simulink model "PX4_Run_Mode_R2016b"  (R2017b)
settings: Solver=FixedStepDiscrete  StartTime=0.0  StopTime=inf  FixedStep=Ts  RelTol=1e-3  EnableMultiTasking=on
InitFcn:
  | run('InitFcn_R2016b.m');
values from neighbouring files (symbols this model uses):
  A = Pixhawk_CSC.Parameter( {single([diag([1 1 1]) Ts*diag([1 1 1]); diag([0 0 0]) diag([1 1 1])]),'A'} )    [InitFcn.m]    (also in InitFcn_R2016b.m; InitFcn_R2017b_no_csc.m = single([diag([1 1 1]) Ts*diag([1 1 1]); diag([0 0 0]) diag([)
  app = Pixhawk_CSC.Parameter({single( [0.05; 0.05; 0.05]),'app'} )    [InitFcn.m]    (also in InitFcn_R2016b.m; InitFcn_R2017b_no_csc.m = single( [0.05; 0.05; 0.05]))
  B = Pixhawk_CSC.Parameter( {single([Ts^2/2*diag([1 1 1]); Ts*diag([1 1 1])]),'B'} )    [InitFcn.m]    (also in InitFcn_R2016b.m; InitFcn_R2017b_no_csc.m = single([Ts^2/2*diag([1 1 1]); Ts*diag([1 1 1])]))
  Beta = Pixhawk_CSC.Parameter({single( 0.02),'Beta'} )    [InitFcn.m]    (also in InitFcn_R2016b.m; InitFcn_R2017b_no_csc.m = single( 0.02))
  C = Pixhawk_CSC.Parameter( {single([diag([1 1 1]) 0*diag([1 1 1]); zeros(1,2) 1 zeros(1,3)]),'C'} )    [InitFcn.m]    (also in InitFcn_R2016b.m; InitFcn_R2017b_no_csc.m = single([diag([1 1 1]) 0*diag([1 1 1]); zeros(1,2) 1 zeros(1,)
  C1 = Pixhawk_CSC.Parameter({single( 1.08680),'C1'} )    [InitFcn.m]    (also in InitFcn_R2016b.m; InitFcn_R2017b_no_csc.m = single( 1.08680))
  C10 = Pixhawk_CSC.Parameter({single( 0.0000),'C10'} )    [InitFcn.m]    (also in InitFcn_R2016b.m; InitFcn_R2017b_no_csc.m = single( 0.0000))
  C11 = Pixhawk_CSC.Parameter({single(-0.2300),'C11'} )    [InitFcn.m]    (also in InitFcn_R2016b.m; InitFcn_R2017b_no_csc.m = single(-0.2300))
  C12 = Pixhawk_CSC.Parameter({single( 0.0000),'C12'} )    [InitFcn.m]    (also in InitFcn_R2016b.m; InitFcn_R2017b_no_csc.m = single( 0.0000))
  C13 = Pixhawk_CSC.Parameter({single( 0.8000),'C13'} )    [InitFcn.m]    (also in InitFcn_R2016b.m; InitFcn_R2017b_no_csc.m = single( 0.8000))
  C14 = Pixhawk_CSC.Parameter({single( 0.8000),'C14'} )    [InitFcn.m]    (also in InitFcn_R2016b.m; InitFcn_R2017b_no_csc.m = single( 0.8000))
  C15 = Pixhawk_CSC.Parameter({single( 1.73200),'C15'} )    [InitFcn.m]    (also in InitFcn_R2016b.m; InitFcn_R2017b_no_csc.m = single( 1.73200))
  C16 = Pixhawk_CSC.Parameter({single( 0.1000),'C16'} )    [InitFcn.m]    (also in InitFcn_R2016b.m; InitFcn_R2017b_no_csc.m = single( 0.1000))
  C17 = Pixhawk_CSC.Parameter({single( 0.1000),'C17'} )    [InitFcn.m]    (also in InitFcn_R2016b.m; InitFcn_R2017b_no_csc.m = single( 0.1000))
  C18 = Pixhawk_CSC.Parameter({single( 0.0500),'C18'} )    [InitFcn.m]    (also in InitFcn_R2016b.m; InitFcn_R2017b_no_csc.m = single( 0.0500))
  C19 = Pixhawk_CSC.Parameter({single( 0.6000),'C19'} )    [InitFcn.m]    (also in InitFcn_R2016b.m; InitFcn_R2017b_no_csc.m = single( 0.6000))
  C2 = Pixhawk_CSC.Parameter({single( 1.10468),'C2'} )    [InitFcn.m]    (also in InitFcn_R2016b.m; InitFcn_R2017b_no_csc.m = single( 1.10468))
  C20 = Pixhawk_CSC.Parameter({single( 0.6000),'C20'} )    [InitFcn.m]    (also in InitFcn_R2016b.m; InitFcn_R2017b_no_csc.m = single( 0.6000))
  C21 = Pixhawk_CSC.Parameter({single( 1.04558),'C21'} )    [InitFcn.m]    (also in InitFcn_R2016b.m; InitFcn_R2017b_no_csc.m = single( 1.04558))
  C22 = Pixhawk_CSC.Parameter({single( 0.0000),'C22'} )    [InitFcn.m]    (also in InitFcn_R2016b.m; InitFcn_R2017b_no_csc.m = single( 0.0000))
  C23 = Pixhawk_CSC.Parameter({single( 0.0000),'C23'} )    [InitFcn.m]    (also in InitFcn_R2016b.m; InitFcn_R2017b_no_csc.m = single( 0.0000))
  C24 = Pixhawk_CSC.Parameter({single(-11.0000),'C24'} )    [InitFcn.m]    (also in InitFcn_R2016b.m; InitFcn_R2017b_no_csc.m = single(-11.0000))
  C3 = Pixhawk_CSC.Parameter({single( 1.1980),'C3'} )    [InitFcn.m]    (also in InitFcn_R2016b.m; InitFcn_R2017b_no_csc.m = single( 1.1980))
  C4 = Pixhawk_CSC.Parameter({single( 0.0500),'C4'} )    [InitFcn.m]    (also in InitFcn_R2016b.m; InitFcn_R2017b_no_csc.m = single( 0.0500))
  C5 = Pixhawk_CSC.Parameter({single( 0.0500),'C5'} )    [InitFcn.m]    (also in InitFcn_R2016b.m; InitFcn_R2017b_no_csc.m = single( 0.0500))
  C6 = Pixhawk_CSC.Parameter({single( 0.0500),'C6'} )    [InitFcn.m]    (also in InitFcn_R2016b.m; InitFcn_R2017b_no_csc.m = single( 0.0500))
  C7 = Pixhawk_CSC.Parameter({single( 0.35937),'C7'} )    [InitFcn.m]    (also in InitFcn_R2016b.m; InitFcn_R2017b_no_csc.m = single( 0.35937))
  C8 = Pixhawk_CSC.Parameter({single( 0.36528),'C8'} )    [InitFcn.m]    (also in InitFcn_R2016b.m; InitFcn_R2017b_no_csc.m = single( 0.36528))
  C9 = Pixhawk_CSC.Parameter({single( 0.53311),'C9'} )    [InitFcn.m]    (also in InitFcn_R2016b.m; InitFcn_R2017b_no_csc.m = single( 0.53311))
  C_1 = Pixhawk_CSC.Parameter( {single([diag([1 1 1]) 0*diag([1 1 1])]),'C1'} )    [InitFcn.m]    (also in InitFcn_R2016b.m; InitFcn_R2017b_no_csc.m = single([diag([1 1 1]) 0*diag([1 1 1])]))
  CAL_ACC0_XOFFSET = Pixhawk_CSC.Parameter( {single( 0.122052  ),'CAL_ACC0_XOFFSET'} )    [InitFcn.m]    (also in InitFcn_R2016b.m; InitFcn_R2017b_no_csc.m = single( 0.122052  ))
  CAL_ACC0_XXSCALE = Pixhawk_CSC.Parameter( {single(  1.01218    ),'CAL_ACC0_XXSCALE'} )    [InitFcn.m]    (also in InitFcn_R2016b.m; InitFcn_R2017b_no_csc.m = single(  1.01218    ))
  CAL_ACC0_XYSCALE = Pixhawk_CSC.Parameter( {single( -0.00443301 ),'CAL_ACC0_XYSCALE'} )    [InitFcn.m]    (also in InitFcn_R2016b.m; InitFcn_R2017b_no_csc.m = single( -0.00443301 ))
  CAL_ACC0_XZSCALE = Pixhawk_CSC.Parameter( {single( -0.00505793 ),'CAL_ACC0_XZSCALE'} )    [InitFcn.m]    (also in InitFcn_R2016b.m; InitFcn_R2017b_no_csc.m = single( -0.00505793 ))
  CAL_ACC0_YOFFSET = Pixhawk_CSC.Parameter( {single( 0.00281205),'CAL_ACC0_YOFFSET'} )    [InitFcn.m]    (also in InitFcn_R2016b.m; InitFcn_R2017b_no_csc.m = single( 0.00281205))
  CAL_ACC0_YXSCALE = Pixhawk_CSC.Parameter( {single( -0.00443301 ),'CAL_ACC0_YXSCALE'} )    [InitFcn.m]    (also in InitFcn_R2016b.m; InitFcn_R2017b_no_csc.m = single( -0.00443301 ))
  CAL_ACC0_YYSCALE = Pixhawk_CSC.Parameter( {single(  1.00234    ),'CAL_ACC0_YYSCALE'} )    [InitFcn.m]    (also in InitFcn_R2016b.m; InitFcn_R2017b_no_csc.m = single(  1.00234    ))
  CAL_ACC0_YZSCALE = Pixhawk_CSC.Parameter( {single(  0.0160883  ),'CAL_ACC0_YZSCALE'} )    [InitFcn.m]    (also in InitFcn_R2016b.m; InitFcn_R2017b_no_csc.m = single(  0.0160883  ))
  CAL_ACC0_ZOFFSET = Pixhawk_CSC.Parameter( {single(-0.0298121 ),'CAL_ACC0_ZOFFSET'} )    [InitFcn.m]    (also in InitFcn_R2016b.m; InitFcn_R2017b_no_csc.m = single(-0.0298121 ))
  CAL_ACC0_ZXSCALE = Pixhawk_CSC.Parameter( {single( -0.00505793 ),'CAL_ACC0_ZXSCALE'} )    [InitFcn.m]    (also in InitFcn_R2016b.m; InitFcn_R2017b_no_csc.m = single( -0.00505793 ))
  CAL_ACC0_ZYSCALE = Pixhawk_CSC.Parameter( {single(  0.0160883  ),'CAL_ACC0_ZYSCALE'} )    [InitFcn.m]    (also in InitFcn_R2016b.m; InitFcn_R2017b_no_csc.m = single(  0.0160883  ))
  CAL_ACC0_ZZSCALE = Pixhawk_CSC.Parameter( {single(  0.983604   ),'CAL_ACC0_ZZSCALE'} )    [InitFcn.m]    (also in InitFcn_R2016b.m; InitFcn_R2017b_no_csc.m = single(  0.983604   ))
  CAL_BAR_OFFSET = Pixhawk_CSC.Parameter( {single( -20.8468),'CAL_BAR_OFFSET'} )    [InitFcn.m]    (also in InitFcn_R2016b.m; InitFcn_R2017b_no_csc.m = single( -20.8468))
  CAL_BAR_SCALE = Pixhawk_CSC.Parameter( {single(   1.0632),'CAL_BAR_SCALE'} )    [InitFcn.m]    (also in InitFcn_R2016b.m; InitFcn_R2017b_no_csc.m = single(   1.0632))
  CAL_BAT0_XOFFSET = Pixhawk_CSC.Parameter( {single( 0.0000),'CAL_BAT0_XOFFSET'} )    [InitFcn.m]    (also in InitFcn_R2016b.m; InitFcn_R2017b_no_csc.m = single( 0.0000))
  CAL_BAT0_XXSCALE = Pixhawk_CSC.Parameter( {single(  1.0000),'CAL_BAT0_XXSCALE'} )    [InitFcn.m]    (also in InitFcn_R2016b.m; InitFcn_R2017b_no_csc.m = single(  1.0000))
  CAL_BAT0_XYSCALE = Pixhawk_CSC.Parameter( {single(  0.0000),'CAL_BAT0_XYSCALE'} )    [InitFcn.m]    (also in InitFcn_R2016b.m; InitFcn_R2017b_no_csc.m = single(  0.0000))
  CAL_BAT0_XZSCALE = Pixhawk_CSC.Parameter( {single(  0.0000),'CAL_BAT0_XZSCALE'} )    [InitFcn.m]    (also in InitFcn_R2016b.m; InitFcn_R2017b_no_csc.m = single(  0.0000))
  CAL_BAT0_YOFFSET = Pixhawk_CSC.Parameter( {single( 0.0000),'CAL_BAT0_YOFFSET'} )    [InitFcn.m]    (also in InitFcn_R2016b.m; InitFcn_R2017b_no_csc.m = single( 0.0000))
  CAL_BAT0_YXSCALE = Pixhawk_CSC.Parameter( {single(  0.0000),'CAL_BAT0_YXSCALE'} )    [InitFcn.m]    (also in InitFcn_R2016b.m; InitFcn_R2017b_no_csc.m = single(  0.0000))
  CAL_BAT0_YYSCALE = Pixhawk_CSC.Parameter( {single(  1.0000),'CAL_BAT0_YYSCALE'} )    [InitFcn.m]    (also in InitFcn_R2016b.m; InitFcn_R2017b_no_csc.m = single(  1.0000))
  CAL_BAT0_YZSCALE = Pixhawk_CSC.Parameter( {single(  0.0000),'CAL_BAT0_YZSCALE'} )    [InitFcn.m]    (also in InitFcn_R2016b.m; InitFcn_R2017b_no_csc.m = single(  0.0000))
  CAL_BAT0_ZOFFSET = Pixhawk_CSC.Parameter( {single( 0.0000),'CAL_BAT0_ZOFFSET'} )    [InitFcn.m]    (also in InitFcn_R2016b.m; InitFcn_R2017b_no_csc.m = single( 0.0000))
  CAL_BAT0_ZXSCALE = Pixhawk_CSC.Parameter( {single(  0.0000),'CAL_BAT0_ZXSCALE'} )    [InitFcn.m]    (also in InitFcn_R2016b.m; InitFcn_R2017b_no_csc.m = single(  0.0000))
  CAL_BAT0_ZYSCALE = Pixhawk_CSC.Parameter( {single(  0.0000),'CAL_BAT0_ZYSCALE'} )    [InitFcn.m]    (also in InitFcn_R2016b.m; InitFcn_R2017b_no_csc.m = single(  0.0000))
  CAL_BAT0_ZZSCALE = Pixhawk_CSC.Parameter( {single(  1.0000),'CAL_BAT0_ZZSCALE'} )    [InitFcn.m]    (also in InitFcn_R2016b.m; InitFcn_R2017b_no_csc.m = single(  1.0000))
  CAL_GPS0_XOFFSET = Pixhawk_CSC.Parameter( {single( 0.0000),'CAL_GPS0_XOFFSET'} )    [InitFcn.m]    (also in InitFcn_R2016b.m; InitFcn_R2017b_no_csc.m = single( 0.0000))
  CAL_GPS0_XXSCALE = Pixhawk_CSC.Parameter( {single(  0.0100),'CAL_GPS0_XXSCALE'} )    [InitFcn.m]    (also in InitFcn_R2016b.m; InitFcn_R2017b_no_csc.m = single(  0.0100))
  CAL_GPS0_XYSCALE = Pixhawk_CSC.Parameter( {single(  0.0000),'CAL_GPS0_XYSCALE'} )    [InitFcn.m]    (also in InitFcn_R2016b.m; InitFcn_R2017b_no_csc.m = single(  0.0000))
  CAL_GPS0_XZSCALE = Pixhawk_CSC.Parameter( {single(  0.0000),'CAL_GPS0_XZSCALE'} )    [InitFcn.m]    (also in InitFcn_R2016b.m; InitFcn_R2017b_no_csc.m = single(  0.0000))
  CAL_GPS0_YOFFSET = Pixhawk_CSC.Parameter( {single( 0.0000),'CAL_GPS0_YOFFSET'} )    [InitFcn.m]    (also in InitFcn_R2016b.m; InitFcn_R2017b_no_csc.m = single( 0.0000))
  CAL_GPS0_YXSCALE = Pixhawk_CSC.Parameter( {single(  0.0000),'CAL_GPS0_YXSCALE'} )    [InitFcn.m]    (also in InitFcn_R2016b.m; InitFcn_R2017b_no_csc.m = single(  0.0000))
  CAL_GPS0_YYSCALE = Pixhawk_CSC.Parameter( {single(  0.0100),'CAL_GPS0_YYSCALE'} )    [InitFcn.m]    (also in InitFcn_R2016b.m; InitFcn_R2017b_no_csc.m = single(  0.0100))
  CAL_GPS0_YZSCALE = Pixhawk_CSC.Parameter( {single(  0.0000),'CAL_GPS0_YZSCALE'} )    [InitFcn.m]    (also in InitFcn_R2016b.m; InitFcn_R2017b_no_csc.m = single(  0.0000))
  CAL_GPS0_ZOFFSET = Pixhawk_CSC.Parameter( {single( 0.0000),'CAL_GPS0_ZOFFSET'} )    [InitFcn.m]    (also in InitFcn_R2016b.m; InitFcn_R2017b_no_csc.m = single( 0.0000))
  CAL_GPS0_ZXSCALE = Pixhawk_CSC.Parameter( {single(  0.0000),'CAL_GPS0_ZXSCALE'} )    [InitFcn.m]    (also in InitFcn_R2016b.m; InitFcn_R2017b_no_csc.m = single(  0.0000))
  CAL_GPS0_ZYSCALE = Pixhawk_CSC.Parameter( {single(  0.0000),'CAL_GPS0_ZYSCALE'} )    [InitFcn.m]    (also in InitFcn_R2016b.m; InitFcn_R2017b_no_csc.m = single(  0.0000))
  CAL_GPS0_ZZSCALE = Pixhawk_CSC.Parameter( {single( -0.0010),'CAL_GPS0_ZZSCALE'} )    [InitFcn.m]    (also in InitFcn_R2016b.m; InitFcn_R2017b_no_csc.m = single( -0.0010))
  CAL_GYRO0_XXSCALE = Pixhawk_CSC.Parameter( {single(0.992736),'CAL_GYRO0_XXSCALE'} )    [InitFcn.m]    (also in InitFcn_R2016b.m; InitFcn_R2017b_no_csc.m = single(0.992736))
  CAL_GYRO0_XYSCALE = Pixhawk_CSC.Parameter( {single(0.0000),'CAL_GYRO0_XYSCALE'} )    [InitFcn.m]    (also in InitFcn_R2016b.m; InitFcn_R2017b_no_csc.m = single(0.0000))
  CAL_GYRO0_XZSCALE = Pixhawk_CSC.Parameter( {single(0.0000),'CAL_GYRO0_XZSCALE'} )    [InitFcn.m]    (also in InitFcn_R2016b.m; InitFcn_R2017b_no_csc.m = single(0.0000))
  CAL_GYRO0_YXSCALE = Pixhawk_CSC.Parameter( {single(0.0000),'CAL_GYRO0_YXSCALE'} )    [InitFcn.m]    (also in InitFcn_R2016b.m; InitFcn_R2017b_no_csc.m = single(0.0000))
  CAL_GYRO0_YYSCALE = Pixhawk_CSC.Parameter( {single(1.01609),'CAL_GYRO0_YYSCALE'} )    [InitFcn.m]    (also in InitFcn_R2016b.m; InitFcn_R2017b_no_csc.m = single(1.01609))
  CAL_GYRO0_YZSCALE = Pixhawk_CSC.Parameter( {single(0.0000),'CAL_GYRO0_YZSCALE'} )    [InitFcn.m]    (also in InitFcn_R2016b.m; InitFcn_R2017b_no_csc.m = single(0.0000))
  CAL_GYRO0_ZXSCALE = Pixhawk_CSC.Parameter( {single(0.0000),'CAL_GYRO0_ZXSCALE'} )    [InitFcn.m]    (also in InitFcn_R2016b.m; InitFcn_R2017b_no_csc.m = single(0.0000))
  CAL_GYRO0_ZYSCALE = Pixhawk_CSC.Parameter( {single(0.0000),'CAL_GYRO0_ZYSCALE'} )    [InitFcn.m]    (also in InitFcn_R2016b.m; InitFcn_R2017b_no_csc.m = single(0.0000))
  CAL_GYRO0_ZZSCALE = Pixhawk_CSC.Parameter( {single(1.03003),'CAL_GYRO0_ZZSCALE'} )    [InitFcn.m]    (also in InitFcn_R2016b.m; InitFcn_R2017b_no_csc.m = single(1.03003))
  CAL_MAG0_XCURCOR = Pixhawk_CSC.Parameter( {single( 0.0017     ),'CAL_MAG0_XCURCOR'} )    [InitFcn.m]    (also in InitFcn_R2016b.m; InitFcn_R2017b_no_csc.m = single( 0.0017     ))
  CAL_MAG0_XOFFSET = Pixhawk_CSC.Parameter( {single( 0.0446372  ),'CAL_MAG0_XOFFSET'} )    [InitFcn.m]    (also in InitFcn_R2016b.m; InitFcn_R2017b_no_csc.m = single( 0.0446372  ))
  CAL_MAG0_XXSCALE = Pixhawk_CSC.Parameter( {single(  1.01563   ),'CAL_MAG0_XXSCALE'} )    [InitFcn.m]    (also in InitFcn_R2016b.m; InitFcn_R2017b_no_csc.m = single(  1.01563   ))
  CAL_MAG0_XYSCALE = Pixhawk_CSC.Parameter( {single( -0.0612061 ),'CAL_MAG0_XYSCALE'} )    [InitFcn.m]    (also in InitFcn_R2016b.m; InitFcn_R2017b_no_csc.m = single( -0.0612061 ))
  CAL_MAG0_XZSCALE = Pixhawk_CSC.Parameter( {single( -0.011532  ),'CAL_MAG0_XZSCALE'} )    [InitFcn.m]    (also in InitFcn_R2016b.m; InitFcn_R2017b_no_csc.m = single( -0.011532  ))
  CAL_MAG0_YCURCOR = Pixhawk_CSC.Parameter( {single(-0.0075     ),'CAL_MAG0_YCURCOR'} )    [InitFcn.m]    (also in InitFcn_R2016b.m; InitFcn_R2017b_no_csc.m = single(-0.0075     ))
  CAL_MAG0_YOFFSET = Pixhawk_CSC.Parameter( {single( 0.0700776  ),'CAL_MAG0_YOFFSET'} )    [InitFcn.m]    (also in InitFcn_R2016b.m; InitFcn_R2017b_no_csc.m = single( 0.0700776  ))
  CAL_MAG0_YXSCALE = Pixhawk_CSC.Parameter( {single( -0.0612061 ),'CAL_MAG0_YXSCALE'} )    [InitFcn.m]    (also in InitFcn_R2016b.m; InitFcn_R2017b_no_csc.m = single( -0.0612061 ))
  CAL_MAG0_YYSCALE = Pixhawk_CSC.Parameter( {single(  1.00593   ),'CAL_MAG0_YYSCALE'} )    [InitFcn.m]    (also in InitFcn_R2016b.m; InitFcn_R2017b_no_csc.m = single(  1.00593   ))
  CAL_MAG0_YZSCALE = Pixhawk_CSC.Parameter( {single(  0.0144582 ),'CAL_MAG0_YZSCALE'} )    [InitFcn.m]    (also in InitFcn_R2016b.m; InitFcn_R2017b_no_csc.m = single(  0.0144582 ))
  CAL_MAG0_ZCURCOR = Pixhawk_CSC.Parameter( {single(-0.0080     ),'CAL_MAG0_ZCURCOR'} )    [InitFcn.m]    (also in InitFcn_R2016b.m; InitFcn_R2017b_no_csc.m = single(-0.0080     ))
  CAL_MAG0_ZOFFSET = Pixhawk_CSC.Parameter( {single( 0.00201742 ),'CAL_MAG0_ZOFFSET'} )    [InitFcn.m]    (also in InitFcn_R2016b.m; InitFcn_R2017b_no_csc.m = single( 0.00201742 ))
  CAL_MAG0_ZXSCALE = Pixhawk_CSC.Parameter( {single( -0.011532  ),'CAL_MAG0_ZXSCALE'} )    [InitFcn.m]    (also in InitFcn_R2016b.m; InitFcn_R2017b_no_csc.m = single( -0.011532  ))
  CAL_MAG0_ZYSCALE = Pixhawk_CSC.Parameter( {single(  0.0144582 ),'CAL_MAG0_ZYSCALE'} )    [InitFcn.m]    (also in InitFcn_R2016b.m; InitFcn_R2017b_no_csc.m = single(  0.0144582 ))
  CAL_MAG0_ZZSCALE = Pixhawk_CSC.Parameter( {single(  0.986813  ),'CAL_MAG0_ZZSCALE'} )    [InitFcn.m]    (also in InitFcn_R2016b.m; InitFcn_R2017b_no_csc.m = single(  0.986813  ))
  CAL_SONAR_OFFSET = Pixhawk_CSC.Parameter( {single( -6.8730),'CAL_SONAR_OFFSET'} )    [InitFcn.m]    (also in InitFcn_R2016b.m; InitFcn_R2017b_no_csc.m = single( -6.8730))
  CAL_SONAR_SCALE = Pixhawk_CSC.Parameter( {single(-438.1875),'CAL_SONAR_SCALE'} )    [InitFcn.m]    (also in InitFcn_R2016b.m; InitFcn_R2017b_no_csc.m = single(-438.1875))
  COM_RATE = double(10)    [InitFcn.m]    (also in InitFcn_R2016b.m; InitFcn_R2017b_no_csc.m)
  D = Pixhawk_CSC.Parameter( {single(zeros(size(C.Value,1), size(B.Value,2))),'D'} )    [InitFcn.m]    (also in InitFcn_R2016b.m; InitFcn_R2017b_no_csc.m = single(zeros(size(C,1), size(B,2))))
  Dip0 = Pixhawk_CSC.Parameter({single( 1.2),'Dip0'} )    [InitFcn.m]    (also in InitFcn_R2016b.m; InitFcn_R2017b_no_csc.m = single( 1.2))
  I = Pixhawk_CSC.Parameter( {single(eye(size(Q.Value))),'I'} )    [InitFcn.m]    (also in InitFcn_R2016b.m; InitFcn_R2017b_no_csc.m = single(eye(size(Q))))
  Jxx = Pixhawk_CSC.Parameter( {single(J(1,1)),'Jxx'} )    [InitFcn.m]    (also in InitFcn_R2016b.m; InitFcn_R2017b_no_csc.m = single(J(1,1)))
  Jyy = Pixhawk_CSC.Parameter( {single(J(2,2)),'Jyy'} )    [InitFcn.m]    (also in InitFcn_R2016b.m; InitFcn_R2017b_no_csc.m = single(J(2,2)))
  Jzz = Pixhawk_CSC.Parameter( {single(J(3,3)),'Jzz'} )    [InitFcn.m]    (also in InitFcn_R2016b.m; InitFcn_R2017b_no_csc.m = single(J(3,3)))
  Kapp = Pixhawk_CSC.Parameter({single( 1.2),'Kapp'} )    [InitFcn.m]    (also in InitFcn_R2016b.m; InitFcn_R2017b_no_csc.m = single( 1.2))
  Kx = Pixhawk_CSC.Parameter({single( Kx),'Kx'} )    [InitFcn.m]    (also in InitFcn_R2016b.m = Pixhawk_CSC.Parameter({single( [0.60 0.9]),'Kx'} ); InitFcn_R2017b_no_csc.m = single( [0.60 0.9]))
  Ky = Pixhawk_CSC.Parameter({single( Ky),'Ky'} )    [InitFcn.m]    (also in InitFcn_R2016b.m = Pixhawk_CSC.Parameter({single( [0.4 0.9]),'Ky'} ); InitFcn_R2017b_no_csc.m = single( [0.4 0.9]))
  LPF_REF_DEN = Pixhawk_CSC.Parameter( {single([1.0000 -0.8187]),'LPF_REF_DEN'} )    [InitFcn.m]    (also in InitFcn_R2016b.m; InitFcn_R2017b_no_csc.m = single([1.0000 -0.8187]))
  LPF_REF_NUM = Pixhawk_CSC.Parameter( {single([0.0000  0.1813]),'LPF_REF_NUM'} )    [InitFcn.m]    (also in InitFcn_R2016b.m; InitFcn_R2017b_no_csc.m = single([0.0000  0.1813]))
  m0 = Pixhawk_CSC.Parameter({single( 0.452857),'m0'} )    [InitFcn.m]    (also in InitFcn_R2016b.m; InitFcn_R2017b_no_csc.m = single( 0.452857))
  mn = [0.01; 0.01; 0.01; 0.01]    [InitFcn.m]    (also in InitFcn_R2016b.m; InitFcn_R2017b_no_csc.m)
  MOV_AVG_WINDOW = Pixhawk_CSC.Parameter( {single(100),'MOV_AVG_WINDOW'} )    [InitFcn.m]    (also in InitFcn_R2016b.m; InitFcn_R2017b_no_csc.m = single(100))
  Ox0 = Pixhawk_CSC.Parameter({single(O_x0),'Ox0'} )    [InitFcn.m]    (also in InitFcn_R2016b.m; InitFcn_R2017b_no_csc.m = single(O_x0))
  Oxa = Pixhawk_CSC.Parameter({single(O_x.a),'Oxa'} )    [InitFcn.m]    (also in InitFcn_R2016b.m; InitFcn_R2017b_no_csc.m = single(O_x.a))
  Oxb = Pixhawk_CSC.Parameter({single(O_x.b),'Oxb'} )    [InitFcn.m]    (also in InitFcn_R2016b.m; InitFcn_R2017b_no_csc.m = single(O_x.b))
  Oxc = Pixhawk_CSC.Parameter({single(O_x.c),'Oxc'} )    [InitFcn.m]    (also in InitFcn_R2016b.m; InitFcn_R2017b_no_csc.m = single(O_x.c))
  Oxd = Pixhawk_CSC.Parameter({single(O_x.d),'Oxd'} )    [InitFcn.m]    (also in InitFcn_R2016b.m; InitFcn_R2017b_no_csc.m = single(O_x.d))
  Oy0 = Pixhawk_CSC.Parameter({single(O_y0),'Oy0'} )    [InitFcn.m]    (also in InitFcn_R2016b.m; InitFcn_R2017b_no_csc.m = single(O_y0))
  Oya = Pixhawk_CSC.Parameter({single(O_y.a),'Oya'} )    [InitFcn.m]    (also in InitFcn_R2016b.m; InitFcn_R2017b_no_csc.m = single(O_y.a))
  Oyb = Pixhawk_CSC.Parameter({single(O_y.b),'Oyb'} )    [InitFcn.m]    (also in InitFcn_R2016b.m; InitFcn_R2017b_no_csc.m = single(O_y.b))
  Oyc = Pixhawk_CSC.Parameter({single(O_y.c),'Oyc'} )    [InitFcn.m]    (also in InitFcn_R2016b.m; InitFcn_R2017b_no_csc.m = single(O_y.c))
  Oyd = Pixhawk_CSC.Parameter({single(O_y.d),'Oyd'} )    [InitFcn.m]    (also in InitFcn_R2016b.m; InitFcn_R2017b_no_csc.m = single(O_y.d))
  Oz0 = Pixhawk_CSC.Parameter({single(O_z0),'Oz0'} )    [InitFcn.m]    (also in InitFcn_R2016b.m; InitFcn_R2017b_no_csc.m = single(O_z0))
  ... (+53 more)
undefined symbols (not defined in the file or in its folder): AccX, AccY, AccZ, Altitude, ax, ay, az, Current, FILTER_N, GPS_TS, GyroX, GyroY, GyroZ, Latitude, Longitude, M1_PWM, M2_PWM, M3_PWM, M4_PWM, MagX, MagY, MagZ, mAH, MOTOR, phi, Position_TS, psi, PX4_TUNE_ENUM, RGBLED_COLOR_ENUM, RGBLED_MODE_ENUM, S_AccX, S_AccY, S_AccZ, S_Altitude, S_Baro, S_Current, S_GyroX, S_GyroY, S_GyroZ, S_Latitude, S_Longitude, S_MagX, S_MagY, S_MagZ, S_mAH, S_N_Sat, S_Voltage, T_PITCH, T_ROLL, T_THROTTLE, theta, v, Voltage, w, wx, wxd, wy, wyd, wz ... (+4)
libraries: simulink x31, pixhawk_slib_sensors_actuators x7, pixhawk_slib_ADC_serial x5, pixhawk_slib_misc_utils x3, etargetslib x2
(part 4 of 7)

== system PX4_Run_Mode_R2016b/CONTROLLER/Outer Control Loop/X Control ==
  ERROR_IN : Inport
  TARGET : Inport  Port=2
  ESTIMATED_STATE_IN : Inport  Port=3
  SYSTEM_MODE_IN : Inport  Port=4
  Add : Sum
  Add2 : Sum  Inputs=+-
  Add4 : Sum  Inputs=-+
  Bus Assignment : BusAssignment  AssignedSignals=e16,e17,e18,e19,e20
  Bus Selector1 : BusSelector  OutputSignals=x,u
  Bus Selector2 : BusSelector  OutputSignals=ARM_CMD,AUTO_FLIGHT
  Bus Selector3 : BusSelector  OutputSignals=T_X
  Constant1 : Constant  Value=0  SampleTime=Ts
  Constant2 : Constant  Value=0  SampleTime=Ts
  D Controller : simulink/Continuous/PID Controller  Controller=PID  TimeDomain=Discrete-time  SampleTime=Ts  IntegratorMethod=Forward Euler  FilterMethod=Forward Euler  Form=Parallel  UseFilter=on  ControllerParametersSource=internal  P=Kx(2)  I=0  D=0  N=100  InitialConditionSource=internal  InitialConditionForIntegrator=0  InitialConditionForFilter=0  ExternalReset=level  LimitOutput=off  UpperSaturationLimit=0.25  LowerSaturationLimit=-0.25  LinearizeAsGain=on  AntiWindupMode=clamping  Kb=1  TrackingMode=off  Kt=1  PParamMin=[]  PParamMax=[]  PParamDataTypeStr=single  IParamMin=[]  IParamMax=[]  IParamDataTypeStr=single  DParamMin=[]  DParamMax=[]  DParamDataTypeStr=single  NParamMin=[]  NParamMax=[]  NParamDataTypeStr=single  KbParamMin=[]  KbParamMax=[]  KtParamMin=[]  KtParamMax=[]  POutMin=[]  POutMax=[]  POutDataTypeStr=single  PGainOutDataTypeStr=single  PProdOutDataTypeStr=single  IOutMin=[]  IOutMax=[]  IOutDataTypeStr=single  IGainOutDataTypeStr=single  IProdOutDataTypeStr=single  DOutMin=[]  DOutMax=[]  DOutDataTypeStr=single  DGainOutDataTypeStr=single  DProdOutDataTypeStr=single  NOutMin=[]  NOutMax=[]  NOutDataTypeStr=single  NGainOutDataTypeStr=single  NProdOutDataTypeStr=single  KbOutMin=[]  KbOutMax=[]  KtOutMin=[]  KtOutMax=[]  IntegratorOutMin=[]  IntegratorOutMax=[]  IntegratorOutDataTypeStr=single  FilterOutMin=[]  FilterOutMax=[]  FilterOutDataTypeStr=single  SumOutMin=[]  SumOutMax=[]  SumOutDataTypeStr=single  SumI1OutMin=[]  SumI1OutMax=[]  SumI2OutMin=[]  SumI2OutMax=[]  SumI3OutMin=[]  SumI3OutMax=[]  SumDOutMin=[]  SumDOutMax=[]  SumDOutDataTypeStr=single  SumAccumDataTypeStr=single  SumDAccumDataTypeStr=single  SaturationOutMin=[]  SaturationOutMax=[]  IntegratorContinuousStateAttributes=''  IntegratorStateMustResolveToSignalObject=off  IntegratorRTWStateStorageClass=Auto  FilterContinuousStateAttributes=''  FilterStateMustResolveToSignalObject=off  FilterRTWStateStorageClass=Auto  DifferentiatorICPrevScaledInput=0  DifferentiatorOutMin=[]  DifferentiatorOutMax=[]  InitialConditionSetting=State (most efficient)  FilterDiffOutCoefMin=[]  FilterDiffOutCoefMax=[]  SumDenOutMin=[]  SumDenOutMax=[]  SumNumOutMin=[]  SumNumOutMax=[]  ReciprocalOutMin=[]  ReciprocalOutMax=[]  DivideOutMin=[]  DivideOutMax=[]  TunerSelectOption=Transfer Function Based (PID Tuner App)
  Data Type Conversion1 : DataTypeConversion  OutDataTypeStr=single
  Data Type Conversion2 : DataTypeConversion  OutDataTypeStr=single
  Logical Operator : Logic  IconShape=distinctive  AllPortsSameDT=off  OutDataTypeStr=boolean
  Logical Operator1 : Logic  Operator=NOT  IconShape=distinctive  AllPortsSameDT=off  OutDataTypeStr=boolean
  PI Controller : simulink/Continuous/PID Controller  Controller=PID  TimeDomain=Discrete-time  SampleTime=Ts  IntegratorMethod=Forward Euler  FilterMethod=Forward Euler  Form=Parallel  UseFilter=on  ControllerParametersSource=internal  P=Kx(1)  I=0  D=0  N=100  InitialConditionSource=internal  InitialConditionForIntegrator=0  InitialConditionForFilter=0  ExternalReset=level  LimitOutput=off  UpperSaturationLimit=0.25  LowerSaturationLimit=-0.25  LinearizeAsGain=on  AntiWindupMode=clamping  Kb=1  TrackingMode=off  Kt=1  PParamMin=[]  PParamMax=[]  PParamDataTypeStr=single  IParamMin=[]  IParamMax=[]  IParamDataTypeStr=single  DParamMin=[]  DParamMax=[]  DParamDataTypeStr=single  NParamMin=[]  NParamMax=[]  NParamDataTypeStr=single  KbParamMin=[]  KbParamMax=[]  KtParamMin=[]  KtParamMax=[]  POutMin=[]  POutMax=[]  POutDataTypeStr=single  PGainOutDataTypeStr=single  PProdOutDataTypeStr=single  IOutMin=[]  IOutMax=[]  IOutDataTypeStr=single  IGainOutDataTypeStr=single  IProdOutDataTypeStr=single  DOutMin=[]  DOutMax=[]  DOutDataTypeStr=single  DGainOutDataTypeStr=single  DProdOutDataTypeStr=single  NOutMin=[]  NOutMax=[]  NOutDataTypeStr=single  NGainOutDataTypeStr=single  NProdOutDataTypeStr=single  KbOutMin=[]  KbOutMax=[]  KtOutMin=[]  KtOutMax=[]  IntegratorOutMin=[]  IntegratorOutMax=[]  IntegratorOutDataTypeStr=single  FilterOutMin=[]  FilterOutMax=[]  FilterOutDataTypeStr=single  SumOutMin=[]  SumOutMax=[]  SumOutDataTypeStr=single  SumI1OutMin=[]  SumI1OutMax=[]  SumI2OutMin=[]  SumI2OutMax=[]  SumI3OutMin=[]  SumI3OutMax=[]  SumDOutMin=[]  SumDOutMax=[]  SumDOutDataTypeStr=single  SumAccumDataTypeStr=single  SumDAccumDataTypeStr=single  SaturationOutMin=[]  SaturationOutMax=[]  SaturationOutDataTypeStr=single  IntegratorContinuousStateAttributes=''  IntegratorStateMustResolveToSignalObject=off  IntegratorRTWStateStorageClass=Auto  FilterContinuousStateAttributes=''  FilterStateMustResolveToSignalObject=off  FilterRTWStateStorageClass=Auto  DifferentiatorICPrevScaledInput=0  DifferentiatorOutMin=[]  DifferentiatorOutMax=[]  InitialConditionSetting=State (most efficient)  FilterDiffOutCoefMin=[]  FilterDiffOutCoefMax=[]  SumDenOutMin=[]  SumDenOutMax=[]  SumNumOutMin=[]  SumNumOutMax=[]  ReciprocalOutMin=[]  ReciprocalOutMax=[]  DivideOutMin=[]  DivideOutMax=[]  TunerSelectOption=Transfer Function Based (PID Tuner App)
  U X : Outport
  ERROR_OUT : Outport  Port=2
  wires:
  ESTIMATED_STATE_IN/1 -> Bus Selector1/1
  TARGET/1 -> Bus Selector3/1
  Bus Assignment/1 -> ERROR_OUT/1
  ERROR_IN/1 -> Bus Assignment/1
  SYSTEM_MODE_IN/1 -> Bus Selector2/1
  Bus Selector2/1 -> Logical Operator/1  "<ARM_CMD>"
  Bus Selector2/2 -> Logical Operator/2  "<AUTO_FLIGHT>"
  Logical Operator/1 -> Logical Operator1/1
  Bus Selector1/2 -> Add4/1  "<u>"
  Logical Operator1/1 -> PI Controller/2, D Controller/2
  PI Controller/1 -> Bus Assignment/3, Add/1
  D Controller/1 -> Bus Assignment/4, Add/2
  Add/1 -> Bus Assignment/6, U X/1
  Add2/1 -> Bus Assignment/2, PI Controller/1
  Bus Selector1/1 -> Add2/2  "<x>"
  Bus Selector3/1 -> Add2/1  "<T_X>"
  Add4/1 -> D Controller/1
  Constant1/1 -> Data Type Conversion1/1
  Data Type Conversion1/1 -> Add4/2
  Constant2/1 -> Data Type Conversion2/1
  Data Type Conversion2/1 -> Bus Assignment/5

== system PX4_Run_Mode_R2016b/CONTROLLER/Outer Control Loop/Y Control ==
  ERROR_IN : Inport
  TARGET : Inport  Port=2
  ESTIMATED_STATE_IN : Inport  Port=3
  SYSTEM_MODE_IN : Inport  Port=4
  Add : Sum
  Add2 : Sum  Inputs=+-
  Add5 : Sum  Inputs=-+
  Bus Assignment : BusAssignment  AssignedSignals=e21,e22,e23,e24,e25
  Bus Selector1 : BusSelector  OutputSignals=y,v
  Bus Selector3 : BusSelector  OutputSignals=ARM_CMD,AUTO_FLIGHT
  Bus Selector4 : BusSelector  OutputSignals=T_Y
  Constant1 : Constant  Value=0  SampleTime=Ts
  Constant2 : Constant  Value=0  SampleTime=Ts
  D Controller : simulink/Continuous/PID Controller  Controller=PID  TimeDomain=Discrete-time  SampleTime=Ts  IntegratorMethod=Forward Euler  FilterMethod=Forward Euler  Form=Parallel  UseFilter=on  ControllerParametersSource=internal  P=Ky(2)  I=0  D=0  N=100  InitialConditionSource=internal  InitialConditionForIntegrator=0  InitialConditionForFilter=0  ExternalReset=level  LimitOutput=off  UpperSaturationLimit=inf  LowerSaturationLimit=-inf  LinearizeAsGain=on  AntiWindupMode=none  Kb=1  TrackingMode=off  Kt=1  PParamMin=[]  PParamMax=[]  PParamDataTypeStr=single  IParamMin=[]  IParamMax=[]  IParamDataTypeStr=single  DParamMin=[]  DParamMax=[]  DParamDataTypeStr=single  NParamMin=[]  NParamMax=[]  NParamDataTypeStr=single  KbParamMin=[]  KbParamMax=[]  KtParamMin=[]  KtParamMax=[]  POutMin=[]  POutMax=[]  POutDataTypeStr=single  PGainOutDataTypeStr=single  PProdOutDataTypeStr=single  IOutMin=[]  IOutMax=[]  IOutDataTypeStr=single  IGainOutDataTypeStr=single  IProdOutDataTypeStr=single  DOutMin=[]  DOutMax=[]  DOutDataTypeStr=single  DGainOutDataTypeStr=single  DProdOutDataTypeStr=single  NOutMin=[]  NOutMax=[]  NOutDataTypeStr=single  NGainOutDataTypeStr=single  NProdOutDataTypeStr=single  KbOutMin=[]  KbOutMax=[]  KtOutMin=[]  KtOutMax=[]  IntegratorOutMin=[]  IntegratorOutMax=[]  IntegratorOutDataTypeStr=single  FilterOutMin=[]  FilterOutMax=[]  FilterOutDataTypeStr=single  SumOutMin=[]  SumOutMax=[]  SumOutDataTypeStr=single  SumI1OutMin=[]  SumI1OutMax=[]  SumI2OutMin=[]  SumI2OutMax=[]  SumI3OutMin=[]  SumI3OutMax=[]  SumDOutMin=[]  SumDOutMax=[]  SumDOutDataTypeStr=single  SumAccumDataTypeStr=single  SumDAccumDataTypeStr=single  SaturationOutMin=[]  SaturationOutMax=[]  IntegratorContinuousStateAttributes=''  IntegratorStateMustResolveToSignalObject=off  IntegratorRTWStateStorageClass=Auto  FilterContinuousStateAttributes=''  FilterStateMustResolveToSignalObject=off  FilterRTWStateStorageClass=Auto  DifferentiatorICPrevScaledInput=0  DifferentiatorOutMin=[]  DifferentiatorOutMax=[]  InitialConditionSetting=State (most efficient)  FilterDiffOutCoefMin=[]  FilterDiffOutCoefMax=[]  SumDenOutMin=[]  SumDenOutMax=[]  SumNumOutMin=[]  SumNumOutMax=[]  ReciprocalOutMin=[]  ReciprocalOutMax=[]  DivideOutMin=[]  DivideOutMax=[]  TunerSelectOption=Transfer Function Based (PID Tuner App)
  Data Type Conversion1 : DataTypeConversion  OutDataTypeStr=single
  Data Type Conversion2 : DataTypeConversion  OutDataTypeStr=single
  Logical Operator2 : Logic  IconShape=distinctive  AllPortsSameDT=off  OutDataTypeStr=boolean
  Logical Operator3 : Logic  Operator=NOT  IconShape=distinctive  AllPortsSameDT=off  OutDataTypeStr=boolean
  PI Controller : simulink/Continuous/PID Controller  Controller=PID  TimeDomain=Discrete-time  SampleTime=Ts  IntegratorMethod=Forward Euler  FilterMethod=Forward Euler  Form=Parallel  UseFilter=on  ControllerParametersSource=internal  P=Ky(1)  I=0  D=0  N=100  InitialConditionSource=internal  InitialConditionForIntegrator=0  InitialConditionForFilter=0  ExternalReset=level  LimitOutput=off  UpperSaturationLimit=0  LowerSaturationLimit=0  LinearizeAsGain=on  AntiWindupMode=clamping  Kb=1  TrackingMode=off  Kt=1  PParamMin=[]  PParamMax=[]  PParamDataTypeStr=single  IParamMin=[]  IParamMax=[]  IParamDataTypeStr=single  DParamMin=[]  DParamMax=[]  DParamDataTypeStr=single  NParamMin=[]  NParamMax=[]  NParamDataTypeStr=single  KbParamMin=[]  KbParamMax=[]  KtParamMin=[]  KtParamMax=[]  POutMin=[]  POutMax=[]  POutDataTypeStr=single  PGainOutDataTypeStr=single  PProdOutDataTypeStr=single  IOutMin=[]  IOutMax=[]  IOutDataTypeStr=single  IGainOutDataTypeStr=single  IProdOutDataTypeStr=single  DOutMin=[]  DOutMax=[]  DOutDataTypeStr=single  DGainOutDataTypeStr=single  DProdOutDataTypeStr=single  NOutMin=[]  NOutMax=[]  NOutDataTypeStr=single  NGainOutDataTypeStr=single  NProdOutDataTypeStr=single  KbOutMin=[]  KbOutMax=[]  KtOutMin=[]  KtOutMax=[]  IntegratorOutMin=[]  IntegratorOutMax=[]  IntegratorOutDataTypeStr=single  FilterOutMin=[]  FilterOutMax=[]  FilterOutDataTypeStr=single  SumOutMin=[]  SumOutMax=[]  SumOutDataTypeStr=single  SumI1OutMin=[]  SumI1OutMax=[]  SumI2OutMin=[]  SumI2OutMax=[]  SumI3OutMin=[]  SumI3OutMax=[]  SumDOutMin=[]  SumDOutMax=[]  SumDOutDataTypeStr=single  SumAccumDataTypeStr=single  SumDAccumDataTypeStr=single  SaturationOutMin=[]  SaturationOutMax=[]  SaturationOutDataTypeStr=single  IntegratorContinuousStateAttributes=''  IntegratorStateMustResolveToSignalObject=off  IntegratorRTWStateStorageClass=Auto  FilterContinuousStateAttributes=''  FilterStateMustResolveToSignalObject=off  FilterRTWStateStorageClass=Auto  DifferentiatorICPrevScaledInput=0  DifferentiatorOutMin=[]  DifferentiatorOutMax=[]  InitialConditionSetting=State (most efficient)  FilterDiffOutCoefMin=[]  FilterDiffOutCoefMax=[]  SumDenOutMin=[]  SumDenOutMax=[]  SumNumOutMin=[]  SumNumOutMax=[]  ReciprocalOutMin=[]  ReciprocalOutMax=[]  DivideOutMin=[]  DivideOutMax=[]  TunerSelectOption=Transfer Function Based (PID Tuner App)
  U Y : Outport
  ERROR_OUT : Outport  Port=2
  wires:
  Bus Assignment/1 -> ERROR_OUT/1
  ERROR_IN/1 -> Bus Assignment/1
  ESTIMATED_STATE_IN/1 -> Bus Selector1/1
  TARGET/1 -> Bus Selector4/1
  SYSTEM_MODE_IN/1 -> Bus Selector3/1
  Bus Selector3/1 -> Logical Operator2/1  "<ARM_CMD>"
  Bus Selector3/2 -> Logical Operator2/2  "<AUTO_FLIGHT>"
  Logical Operator2/1 -> Logical Operator3/1
  Bus Selector1/2 -> Add5/1  "<v>"
  Logical Operator3/1 -> PI Controller/2, D Controller/2
  PI Controller/1 -> Bus Assignment/3, Add/1
  D Controller/1 -> Bus Assignment/4, Add/2
  Add/1 -> Bus Assignment/6, U Y/1
  Add2/1 -> Bus Assignment/2, PI Controller/1
  Bus Selector1/1 -> Add2/2  "<y>"
  Bus Selector4/1 -> Add2/1  "<T_Y>"
  Add5/1 -> D Controller/1
  Constant2/1 -> Data Type Conversion1/1
  Data Type Conversion1/1 -> Add5/2
  Constant1/1 -> Data Type Conversion2/1
  Data Type Conversion2/1 -> Bus Assignment/5

== system PX4_Run_Mode_R2016b/SENSOR_FILTER/Fixed Bias removal and scaling/Accelerometer Calibration ==
  FILTERED_SENSOR_DATA_IN : Inport
  RAW_SENSOR_DATA_IN : Inport  Port=2
  Bus Assignment : BusAssignment  AssignedSignals=AccX,AccY,AccZ
  Bus Selector1 : BusSelector  OutputSignals=S_AccX,S_AccY,S_AccZ  OutputAsBus=on
  Bus to Vector : BusToVector
  Constant1 : Constant  Value=CAL_ACC0_ZYSCALE  SampleTime=Ts
  Constant10 : Constant  Value=CAL_ACC0_ZZSCALE  SampleTime=Ts
  Constant11 : Constant  Value=CAL_ACC0_ZOFFSET  SampleTime=Ts
  Constant12 : Constant  Value=CAL_ACC0_XZSCALE  SampleTime=Ts
  Constant2 : Constant  Value=CAL_ACC0_ZXSCALE  SampleTime=Ts
  Constant3 : Constant  Value=CAL_ACC0_YYSCALE  SampleTime=Ts
  Constant4 : Constant  Value=CAL_ACC0_YZSCALE  SampleTime=Ts
  Constant5 : Constant  Value=CAL_ACC0_XXSCALE  SampleTime=Ts
  Constant6 : Constant  Value=CAL_ACC0_XYSCALE  SampleTime=Ts
  Constant7 : Constant  Value=CAL_ACC0_XOFFSET  SampleTime=Ts
  Constant8 : Constant  Value=CAL_ACC0_YXSCALE  SampleTime=Ts
  Constant9 : Constant  Value=CAL_ACC0_YOFFSET  SampleTime=Ts
  Demux : Demux  Outputs=3
  MATLAB Function : MATLAB Function  TreatAsAtomicUnit=on
  Mux : Mux  Inputs=12
  Parameters : Outport
  FILTERED_SENSOR_DATA_OUT : Outport  Port=2
  wires:
  FILTERED_SENSOR_DATA_IN/1 -> Bus Assignment/1
  Bus Assignment/1 -> FILTERED_SENSOR_DATA_OUT/1
  RAW_SENSOR_DATA_IN/1 -> Bus Selector1/1
  Bus Selector1/1 -> Bus to Vector/1
  Bus to Vector/1 -> MATLAB Function/1(a)
  MATLAB Function/1(acor) -> Demux/1
  Demux/2 -> Bus Assignment/3
  Demux/1 -> Bus Assignment/2
  Demux/3 -> Bus Assignment/4
  Mux/1 -> Parameters/1
  Constant7/1 -> Mux/10
  Constant9/1 -> Mux/11
  Constant11/1 -> Mux/12
  Constant10/1 -> Mux/9
  Constant1/1 -> Mux/8
  Constant2/1 -> Mux/7
  Constant8/1 -> Mux/4
  Constant3/1 -> Mux/5
  Constant4/1 -> Mux/6
  Constant5/1 -> Mux/1
  Constant6/1 -> Mux/2
  Constant12/1 -> Mux/3

== system PX4_Run_Mode_R2016b/SENSOR_FILTER/Fixed Bias removal and scaling/Barometer Calibration ==
  FILTERED_SENSOR_DATA_IN : Inport
  RAW_SENSOR_DATA_IN : Inport  Port=2
  Bus Assignment : BusAssignment  AssignedSignals=Bar
  Bus Selector2 : BusSelector  OutputSignals=S_Baro  OutputAsBus=on
  Bus to Vector : BusToVector
  Constant5 : Constant  Value=CAL_BAR_SCALE  SampleTime=Ts
  Constant6 : Constant  Value=CAL_BAR_OFFSET  SampleTime=Ts
  MATLAB Function : MATLAB Function  TreatAsAtomicUnit=on
  Mux : Mux  Inputs=2
  Parameters : Outport
  FILTERED_SENSOR_DATA_OUT : Outport  Port=2
  wires:
  FILTERED_SENSOR_DATA_IN/1 -> Bus Assignment/1
  MATLAB Function/1(BAR_Out) -> Bus Assignment/2
  Bus Assignment/1 -> FILTERED_SENSOR_DATA_OUT/1
  RAW_SENSOR_DATA_IN/1 -> Bus Selector2/1
  Bus Selector2/1 -> Bus to Vector/1
  Bus to Vector/1 -> MATLAB Function/1(BAR_In)
  Mux/1 -> Parameters/1
  Constant5/1 -> Mux/1
  Constant6/1 -> Mux/2

== system PX4_Run_Mode_R2016b/SENSOR_FILTER/Fixed Bias removal and scaling/Battery Calibration ==
  FILTERED_SENSOR_DATA_IN : Inport
  RAW_SENSOR_DATA_IN : Inport  Port=2
  Bus Assignment : BusAssignment  AssignedSignals=Voltage,Current,mAH
  Bus Selector2 : BusSelector  OutputSignals=S_Voltage,S_Current,S_mAH  OutputAsBus=on
  Bus to Vector : BusToVector
  Constant1 : Constant  Value=CAL_BAT0_ZYSCALE  SampleTime=Ts
  Constant10 : Constant  Value=CAL_BAT0_ZZSCALE  SampleTime=Ts
  Constant11 : Constant  Value=CAL_BAT0_ZOFFSET  SampleTime=Ts
  Constant12 : Constant  Value=CAL_BAT0_XZSCALE  SampleTime=Ts
  Constant2 : Constant  Value=CAL_BAT0_ZXSCALE  SampleTime=Ts
  Constant3 : Constant  Value=CAL_BAT0_YYSCALE  SampleTime=Ts
  Constant4 : Constant  Value=CAL_BAT0_YZSCALE  SampleTime=Ts
  Constant5 : Constant  Value=CAL_BAT0_XXSCALE  SampleTime=Ts
  Constant6 : Constant  Value=CAL_BAT0_XYSCALE  SampleTime=Ts
  Constant7 : Constant  Value=CAL_BAT0_XOFFSET  SampleTime=Ts
  Constant8 : Constant  Value=CAL_BAT0_YXSCALE  SampleTime=Ts
  Constant9 : Constant  Value=CAL_BAT0_YOFFSET  SampleTime=Ts
  Demux : Demux  Outputs=3
  MATLAB Function : MATLAB Function  TreatAsAtomicUnit=on
  Mux : Mux  Inputs=12
  Parameters : Outport
  FILTERED_SENSOR_DATA_OUT : Outport  Port=2
  wires:
  FILTERED_SENSOR_DATA_IN/1 -> Bus Assignment/1
  Demux/1 -> Bus Assignment/2
  Demux/2 -> Bus Assignment/3
  Demux/3 -> Bus Assignment/4
  Bus Assignment/1 -> FILTERED_SENSOR_DATA_OUT/1
  RAW_SENSOR_DATA_IN/1 -> Bus Selector2/1
  Bus Selector2/1 -> Bus to Vector/1
  Bus to Vector/1 -> MATLAB Function/1(Bat)
  MATLAB Function/1(Batcor) -> Demux/1
  Mux/1 -> Parameters/1
  Constant10/1 -> Mux/9
  Constant1/1 -> Mux/8
  Constant2/1 -> Mux/7
  Constant8/1 -> Mux/4
  Constant3/1 -> Mux/5
  Constant4/1 -> Mux/6
  Constant5/1 -> Mux/1
  Constant6/1 -> Mux/2
  Constant12/1 -> Mux/3
  Constant7/1 -> Mux/10
  Constant9/1 -> Mux/11
  Constant11/1 -> Mux/12

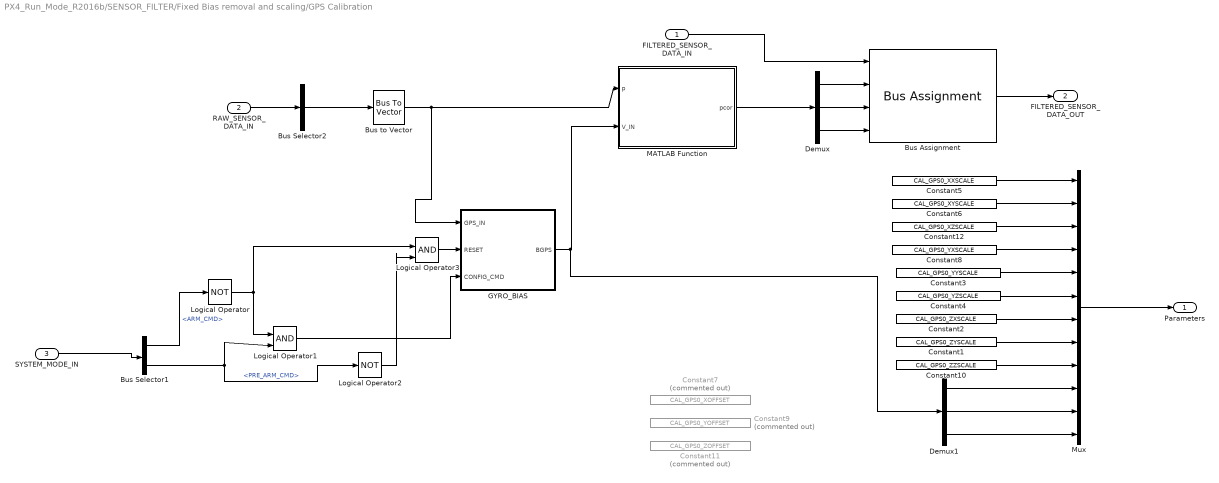
== system PX4_Run_Mode_R2016b/SENSOR_FILTER/Fixed Bias removal and scaling/GPS Calibration ==
  FILTERED_SENSOR_DATA_IN : Inport
  RAW_SENSOR_DATA_IN : Inport  Port=2
  SYSTEM_MODE_IN : Inport  Port=3
  Bus Assignment : BusAssignment  AssignedSignals=Latitude,Longitude,Altitude
  Bus Selector1 : BusSelector  OutputSignals=ARM_CMD,PRE_ARM_CMD
  Bus Selector2 : BusSelector  OutputSignals=S_Latitude,S_Longitude,S_Altitude  OutputAsBus=on
  Bus to Vector : BusToVector
  Constant1 : Constant  Value=CAL_GPS0_ZYSCALE  SampleTime=Ts
  Constant10 : Constant  Value=CAL_GPS0_ZZSCALE  SampleTime=Ts
  Constant11 : Constant  Commented=on  Value=CAL_GPS0_ZOFFSET  SampleTime=Ts
  Constant12 : Constant  Value=CAL_GPS0_XZSCALE  SampleTime=Ts
  Constant2 : Constant  Value=CAL_GPS0_ZXSCALE  SampleTime=Ts
  Constant3 : Constant  Value=CAL_GPS0_YYSCALE  SampleTime=Ts
  Constant4 : Constant  Value=CAL_GPS0_YZSCALE  SampleTime=Ts
  Constant5 : Constant  Value=CAL_GPS0_XXSCALE  SampleTime=Ts
  Constant6 : Constant  Value=CAL_GPS0_XYSCALE  SampleTime=Ts
  Constant7 : Constant  Commented=on  Value=CAL_GPS0_XOFFSET  SampleTime=Ts
  Constant8 : Constant  Value=CAL_GPS0_YXSCALE  SampleTime=Ts
  Constant9 : Constant  Commented=on  Value=CAL_GPS0_YOFFSET  SampleTime=Ts
  Demux : Demux  Outputs=3
  Demux1 : Demux  Outputs=3
  GYRO_BIAS : MATLAB Function  TreatAsAtomicUnit=on
  Logical Operator : Logic  Operator=NOT  IconShape=distinctive  AllPortsSameDT=off  OutDataTypeStr=boolean
  Logical Operator1 : Logic  IconShape=distinctive  AllPortsSameDT=off  OutDataTypeStr=boolean
  Logical Operator2 : Logic  Operator=NOT  IconShape=distinctive  AllPortsSameDT=off  OutDataTypeStr=boolean
  Logical Operator3 : Logic  IconShape=distinctive  AllPortsSameDT=off  OutDataTypeStr=boolean
  MATLAB Function : MATLAB Function  TreatAsAtomicUnit=on
  Mux : Mux  Inputs=12
  Parameters : Outport
  FILTERED_SENSOR_DATA_OUT : Outport  Port=2
  wires:
  FILTERED_SENSOR_DATA_IN/1 -> Bus Assignment/1
  Demux/1 -> Bus Assignment/2
  Demux/2 -> Bus Assignment/3
  Demux/3 -> Bus Assignment/4
  Bus Assignment/1 -> FILTERED_SENSOR_DATA_OUT/1
  RAW_SENSOR_DATA_IN/1 -> Bus Selector2/1
  Bus Selector2/1 -> Bus to Vector/1
  Bus to Vector/1 -> MATLAB Function/1(p), GYRO_BIAS/1(GPS_IN)
  MATLAB Function/1(pcor) -> Demux/1
  Mux/1 -> Parameters/1
  Constant10/1 -> Mux/9
  Constant1/1 -> Mux/8
  Constant2/1 -> Mux/7
  Constant8/1 -> Mux/4
  Constant3/1 -> Mux/5
  Constant4/1 -> Mux/6
  Constant5/1 -> Mux/1
  Constant6/1 -> Mux/2
  Constant12/1 -> Mux/3
  Demux1/1 -> Mux/10
  Demux1/2 -> Mux/11
  Demux1/3 -> Mux/12
  SYSTEM_MODE_IN/1 -> Bus Selector1/1
  Bus Selector1/1 -> Logical Operator/1  "<ARM_CMD>"
  Logical Operator1/1 -> GYRO_BIAS/3(CONFIG_CMD)
  Logical Operator/1 -> Logical Operator1/1, Logical Operator3/1
  Bus Selector1/2 -> Logical Operator2/1, Logical Operator1/2  "<PRE_ARM_CMD>"
  Logical Operator3/1 -> GYRO_BIAS/2(RESET)
  Logical Operator2/1 -> Logical Operator3/2
  GYRO_BIAS/1(BGPS) -> Demux1/1, MATLAB Function/2(V_IN)

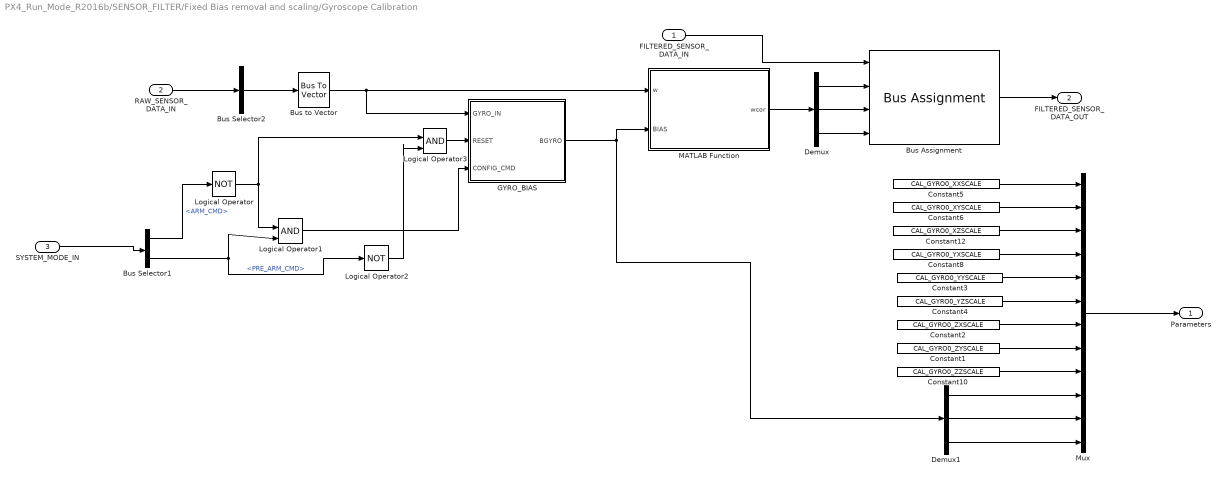
== system PX4_Run_Mode_R2016b/SENSOR_FILTER/Fixed Bias removal and scaling/Gyroscope Calibration ==
  FILTERED_SENSOR_DATA_IN : Inport
  RAW_SENSOR_DATA_IN : Inport  Port=2
  SYSTEM_MODE_IN : Inport  Port=3
  Bus Assignment : BusAssignment  AssignedSignals=GyroX,GyroY,GyroZ
  Bus Selector1 : BusSelector  OutputSignals=ARM_CMD,PRE_ARM_CMD
  Bus Selector2 : BusSelector  OutputSignals=S_GyroX,S_GyroY,S_GyroZ  OutputAsBus=on
  Bus to Vector : BusToVector
  Constant1 : Constant  Value=CAL_GYRO0_ZYSCALE  SampleTime=Ts
  Constant10 : Constant  Value=CAL_GYRO0_ZZSCALE  SampleTime=Ts
  Constant12 : Constant  Value=CAL_GYRO0_XZSCALE  SampleTime=Ts
  Constant2 : Constant  Value=CAL_GYRO0_ZXSCALE  SampleTime=Ts
  Constant3 : Constant  Value=CAL_GYRO0_YYSCALE  SampleTime=Ts
  Constant4 : Constant  Value=CAL_GYRO0_YZSCALE  SampleTime=Ts
  Constant5 : Constant  Value=CAL_GYRO0_XXSCALE  SampleTime=Ts
  Constant6 : Constant  Value=CAL_GYRO0_XYSCALE  SampleTime=Ts
  Constant8 : Constant  Value=CAL_GYRO0_YXSCALE  SampleTime=Ts
  Demux : Demux  Outputs=3
  Demux1 : Demux  Outputs=3
  GYRO_BIAS : MATLAB Function  TreatAsAtomicUnit=on
  Logical Operator : Logic  Operator=NOT  IconShape=distinctive  AllPortsSameDT=off  OutDataTypeStr=boolean
  Logical Operator1 : Logic  IconShape=distinctive  AllPortsSameDT=off  OutDataTypeStr=boolean
  Logical Operator2 : Logic  Operator=NOT  IconShape=distinctive  AllPortsSameDT=off  OutDataTypeStr=boolean
  Logical Operator3 : Logic  IconShape=distinctive  AllPortsSameDT=off  OutDataTypeStr=boolean
  MATLAB Function : MATLAB Function  TreatAsAtomicUnit=on
  Mux : Mux  Inputs=12
  Parameters : Outport
  FILTERED_SENSOR_DATA_OUT : Outport  Port=2
  wires:
  FILTERED_SENSOR_DATA_IN/1 -> Bus Assignment/1
  Demux/1 -> Bus Assignment/2
  Demux/2 -> Bus Assignment/3
  Demux/3 -> Bus Assignment/4
  Bus Assignment/1 -> FILTERED_SENSOR_DATA_OUT/1
  RAW_SENSOR_DATA_IN/1 -> Bus Selector2/1
  Bus Selector2/1 -> Bus to Vector/1
  MATLAB Function/1(wcor) -> Demux/1
  SYSTEM_MODE_IN/1 -> Bus Selector1/1
  Mux/1 -> Parameters/1
  Constant10/1 -> Mux/9
  Constant1/1 -> Mux/8
  Constant2/1 -> Mux/7
  Constant8/1 -> Mux/4
  Constant3/1 -> Mux/5
  Constant4/1 -> Mux/6
  Constant5/1 -> Mux/1
  Constant6/1 -> Mux/2
  Constant12/1 -> Mux/3
  Demux1/3 -> Mux/12
  Demux1/2 -> Mux/11
  Demux1/1 -> Mux/10
  GYRO_BIAS/1(BGYRO) -> Demux1/1, MATLAB Function/2(BIAS)
  Bus to Vector/1 -> GYRO_BIAS/1(GYRO_IN), MATLAB Function/1(w)
  Bus Selector1/1 -> Logical Operator/1  "<ARM_CMD>"
  Logical Operator1/1 -> GYRO_BIAS/3(CONFIG_CMD)
  Logical Operator/1 -> Logical Operator1/1, Logical Operator3/1
  Bus Selector1/2 -> Logical Operator2/1, Logical Operator1/2  "<PRE_ARM_CMD>"
  Logical Operator3/1 -> GYRO_BIAS/2(RESET)
  Logical Operator2/1 -> Logical Operator3/2

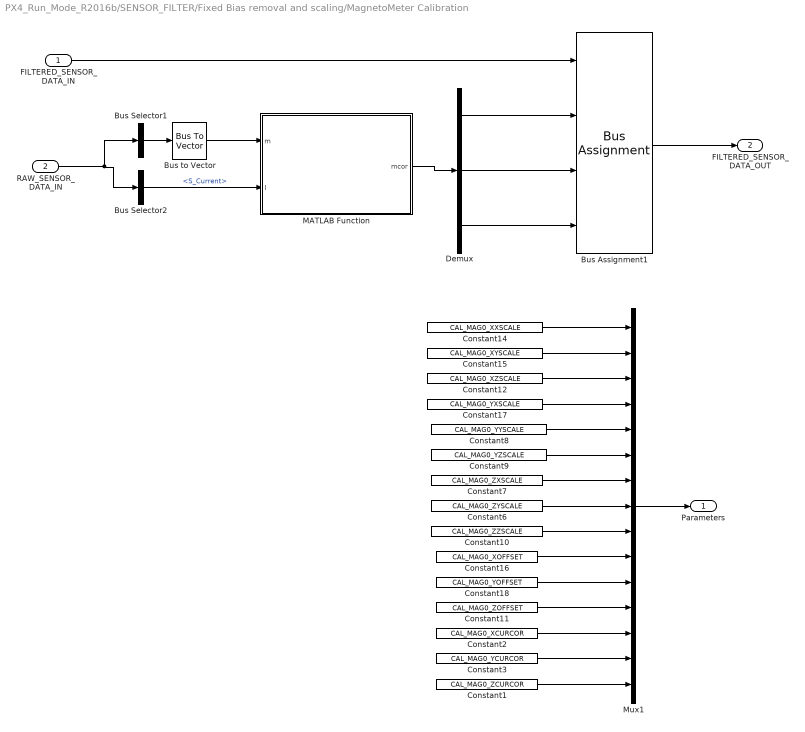
== system PX4_Run_Mode_R2016b/SENSOR_FILTER/Fixed Bias removal and scaling/MagnetoMeter Calibration ==
  FILTERED_SENSOR_DATA_IN : Inport
  RAW_SENSOR_DATA_IN : Inport  Port=2
  Bus Assignment1 : BusAssignment  AssignedSignals=MagX,MagY,MagZ
  Bus Selector1 : BusSelector  OutputSignals=S_MagX,S_MagY,S_MagZ  OutputAsBus=on
  Bus Selector2 : BusSelector  OutputSignals=S_Current
  Bus to Vector : BusToVector
  Constant1 : Constant  Value=CAL_MAG0_ZCURCOR  SampleTime=Ts
  Constant10 : Constant  Value=CAL_MAG0_ZZSCALE  SampleTime=Ts
  Constant11 : Constant  Value=CAL_MAG0_ZOFFSET  SampleTime=Ts
  Constant12 : Constant  Value=CAL_MAG0_XZSCALE  SampleTime=Ts
  Constant14 : Constant  Value=CAL_MAG0_XXSCALE  SampleTime=Ts
  Constant15 : Constant  Value=CAL_MAG0_XYSCALE  SampleTime=Ts
  Constant16 : Constant  Value=CAL_MAG0_XOFFSET  SampleTime=Ts
  Constant17 : Constant  Value=CAL_MAG0_YXSCALE  SampleTime=Ts
  Constant18 : Constant  Value=CAL_MAG0_YOFFSET  SampleTime=Ts
  Constant2 : Constant  Value=CAL_MAG0_XCURCOR  SampleTime=Ts
  Constant3 : Constant  Value=CAL_MAG0_YCURCOR  SampleTime=Ts
  Constant6 : Constant  Value=CAL_MAG0_ZYSCALE  SampleTime=Ts
  Constant7 : Constant  Value=CAL_MAG0_ZXSCALE  SampleTime=Ts
  Constant8 : Constant  Value=CAL_MAG0_YYSCALE  SampleTime=Ts
  Constant9 : Constant  Value=CAL_MAG0_YZSCALE  SampleTime=Ts
  Demux : Demux  Outputs=3
  MATLAB Function : MATLAB Function  TreatAsAtomicUnit=on
  Mux1 : Mux  Inputs=15
  Parameters : Outport
  FILTERED_SENSOR_DATA_OUT : Outport  Port=2
  wires:
  FILTERED_SENSOR_DATA_IN/1 -> Bus Assignment1/1
  Bus Assignment1/1 -> FILTERED_SENSOR_DATA_OUT/1
  RAW_SENSOR_DATA_IN/1 -> Bus Selector2/1, Bus Selector1/1
  Bus Selector1/1 -> Bus to Vector/1
  Bus to Vector/1 -> MATLAB Function/1(m)
  MATLAB Function/1(mcor) -> Demux/1
  Demux/2 -> Bus Assignment1/3
  Demux/1 -> Bus Assignment1/2
  Demux/3 -> Bus Assignment1/4
  Constant16/1 -> Mux1/10
  Constant18/1 -> Mux1/11
  Constant11/1 -> Mux1/12
  Constant10/1 -> Mux1/9
  Constant6/1 -> Mux1/8
  Constant7/1 -> Mux1/7
  Constant17/1 -> Mux1/4
  Constant8/1 -> Mux1/5
  Constant9/1 -> Mux1/6
  Constant14/1 -> Mux1/1
  Constant15/1 -> Mux1/2
  Constant12/1 -> Mux1/3
  Mux1/1 -> Parameters/1
  Constant2/1 -> Mux1/13
  Constant3/1 -> Mux1/14
  Constant1/1 -> Mux1/15
  Bus Selector2/1 -> MATLAB Function/2(I)  "<S_Current>"

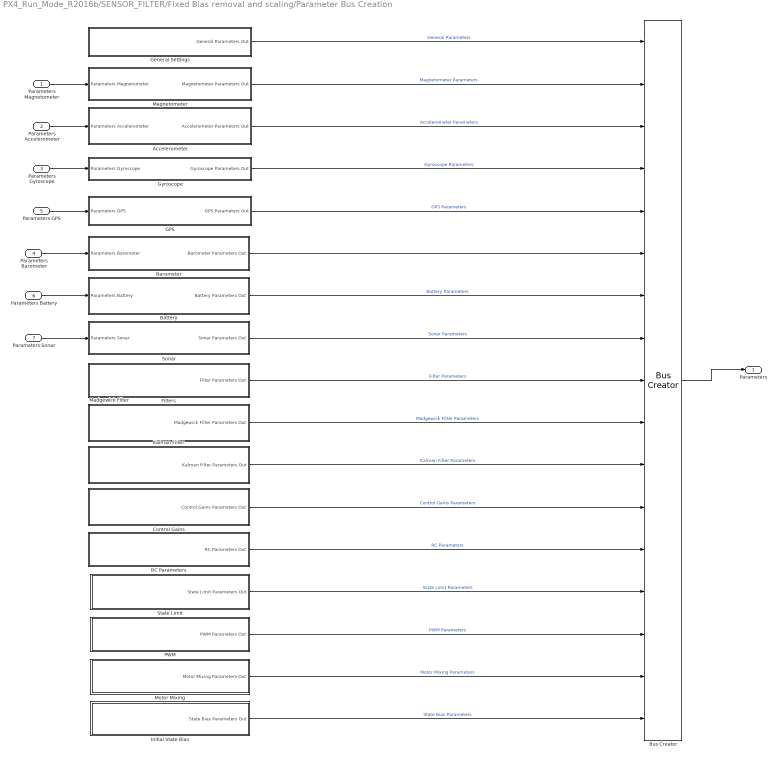
== system PX4_Run_Mode_R2016b/SENSOR_FILTER/Fixed Bias removal and scaling/Parameter Bus Creation ==
  Parameters Magnetometer : Inport
  Parameters Accelerometer : Inport  Port=2
  Parameters Gyroscope : Inport  Port=3
  Parameters Barometer : Inport  Port=4
  Parameters GPS : Inport  Port=5
  Parameters Battery : Inport  Port=6
  Parameters Sonar : Inport  Port=7
  Accelerometer : Subsystem
  Barometer : Subsystem
  Battery : Subsystem
  Bus Creator : BusCreator  Inputs=17
  Control Gains : Subsystem
  Filters : Subsystem
  GPS : Subsystem
  General Settings : Subsystem
  Gyroscope : Subsystem
  Initial State Bias : Subsystem
  Kalman Filter : Subsystem
  Madgewick Filter : Subsystem
  Magnetometer : Subsystem
  Motor Mixing : Subsystem
  PWM : Subsystem
  RC Parameters : Subsystem
  Sonar : Subsystem
  State Limit : Subsystem
  Parameters : Outport
  wires:
  Bus Creator/1 -> Parameters/1
  Control Gains/1(Control Gains Parameters Out) -> Bus Creator/12  "Control Gains Parameters"
  RC Parameters/1(RC Parameters Out) -> Bus Creator/13  "RC Parameters"
  State Limit/1(State Limit Parameters Out) -> Bus Creator/14  "State Limit Parameters"
  PWM/1(PWM Parameters Out) -> Bus Creator/15  "PWM Parameters"
  Motor Mixing/1(Motor Mixing Parameters Out) -> Bus Creator/16  "Motor Mixing Parameters"
  Initial State Bias/1(State Bias Parameters Out) -> Bus Creator/17  "State Bias Parameters"
  Filters/1(Filter Parameters Out) -> Bus Creator/9  "Filter Parameters"
  Parameters Sonar/1 -> Sonar/1(Parameters Sonar)
  Sonar/1(Sonar Parameters Out) -> Bus Creator/8  "Sonar Parameters"
  Parameters Battery/1 -> Battery/1(Parameters Battery)
  Battery/1("Battery Parameters Out ") -> Bus Creator/7  "Battery Parameters"
  Parameters GPS/1 -> GPS/1(Parameters GPS)
  GPS/1(GPS Parameters Out) -> Bus Creator/5  "GPS Parameters"
  Parameters Gyroscope/1 -> Gyroscope/1(Parameters Gyroscope)
  Gyroscope/1(Gyroscope Parameters Out) -> Bus Creator/4  "Gyroscope Parameters"
  Parameters Accelerometer/1 -> Accelerometer/1(Parameters Accelerometer)
  Accelerometer/1(Accelerometer Parameters Out) -> Bus Creator/3  "Accelerometer Parameters"
  Parameters Magnetometer/1 -> Magnetometer/1(Parameters Magnetometer)
  Magnetometer/1(Magnetometer Parameters Out) -> Bus Creator/2  "Magnetometer Parameters"
  General Settings/1(General Parameters Out) -> Bus Creator/1  "General Parameters"
  Kalman Filter/1(Kalman Filter Parameters Out) -> Bus Creator/11  "Kalman Filter Parameters"
  Madgewick Filter/1(Madgewick Filter Parameters Out) -> Bus Creator/10  "Madgewick Filter Parameters"
  Parameters Barometer/1 -> Barometer/1(Parameters Barometer)
  Barometer/1(Barometer Parameters Out) -> Bus Creator/6
